simulink model "WF_status"  (R2022b)
settings: Solver=FixedStepDiscrete  StartTime=0  StopTime=duration  FixedStep=sample_time  RelTol=1e-3
values from neighbouring files (symbols this model uses):
  WF_status_param =     [WF_status_params.mat]
libraries: simulink x6
settings Model: Creator=Carlo_TUM  LastModifiedBy=Carlo_TUM
settings DataIOCC: LoadExternalInput=on  ReturnWorkspaceOutputs=off  ReturnWorkspaceOutputsName=off
settings OptimizationCC: DefaultParameterBehavior=Inlined  EnhancedBackFolding=on  PassReuseOutputArgsAs=Individual arguments  OptimizeBlockOrder=speed  DifferentSizesBufferReuse=on  OptimizationCustomize=off  EfficientTunableParamExpr=on
settings DebuggingCC: ParameterTunabilityLossMsg=error
settings SFSimCC: MATLABDynamicMemAlloc=off
settings RTWCC: Description=Embedded Coder  SystemTargetFile=ert.tlc  TemplateMakefile=ert_default_tmf
settings CodeAppCC: ForceParamTrailComments=on  IgnoreCustomStorageClasses=off  OperatorAnnotations=on  SimulinkDataObjDesc=on  SFDataObjDesc=on  InsertBlockDesc=on
settings ERTTargetCC: TargetLangStandard=C99 (ISO)  GenerateSampleERTMain=on  InlinedParameterPlacement=NonHierarchical  ERTCustomFileTemplate=example_file_process.tlc

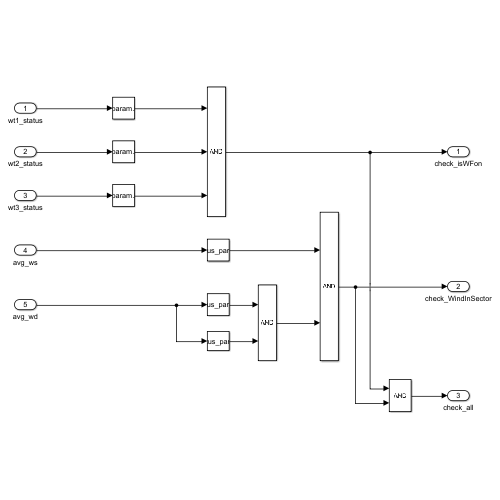
[thumbnail: Simulink's stored preview of the top-level diagram]
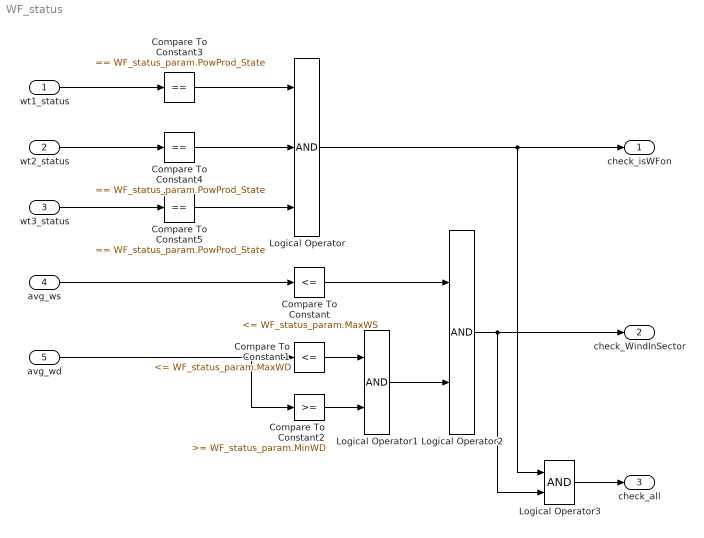
== system WF_status ==
  wt1_status : Inport
  wt2_status : Inport  Port=2
  wt3_status : Inport  Port=3
  avg_ws : Inport  Port=4
  avg_wd : Inport  Port=5
  Compare To Constant : simulink/Logic and Bit Operations/Compare To Constant  relop=<=  const=WF_status_param.MaxWS  OutDataTypeStr=boolean
  Compare To Constant1 : simulink/Logic and Bit Operations/Compare To Constant  relop=<=  const=WF_status_param.MaxWD  OutDataTypeStr=boolean
  Compare To Constant2 : simulink/Logic and Bit Operations/Compare To Constant  relop=>=  const=WF_status_param.MinWD  OutDataTypeStr=boolean
  Compare To Constant3 : simulink/Logic and Bit Operations/Compare To Constant  relop===  const=WF_status_param.PowProd_State  OutDataTypeStr=boolean
  Compare To Constant4 : simulink/Logic and Bit Operations/Compare To Constant  relop===  const=WF_status_param.PowProd_State  OutDataTypeStr=boolean
  Compare To Constant5 : simulink/Logic and Bit Operations/Compare To Constant  relop===  const=WF_status_param.PowProd_State  OutDataTypeStr=boolean
  Logical Operator : Logic  Inputs=3  AllPortsSameDT=off  OutDataTypeStr=boolean
  Logical Operator1 : Logic  AllPortsSameDT=off  OutDataTypeStr=boolean
  Logical Operator2 : Logic  AllPortsSameDT=off  OutDataTypeStr=boolean
  Logical Operator3 : Logic  AllPortsSameDT=off  OutDataTypeStr=boolean
  check_isWFon : Outport
  check_WindInSector : Outport  Port=2
  check_all : Outport  Port=3
  wires:
  wt1_status/1 -> Compare To Constant3/1
  wt2_status/1 -> Compare To Constant4/1
  wt3_status/1 -> Compare To Constant5/1
  Logical Operator/1 -> Logical Operator3/1, check_isWFon/1
  avg_ws/1 -> Compare To Constant/1
  avg_wd/1 -> Compare To Constant2/1, Compare To Constant1/1
  Compare To Constant1/1 -> Logical Operator1/1
  Compare To Constant/1 -> Logical Operator2/1
  Compare To Constant2/1 -> Logical Operator1/2
  Logical Operator1/1 -> Logical Operator2/2
  Logical Operator2/1 -> Logical Operator3/2, check_WindInSector/1
  Logical Operator3/1 -> check_all/1
  Compare To Constant3/1 -> Logical Operator/1
  Compare To Constant4/1 -> Logical Operator/2
  Compare To Constant5/1 -> Logical Operator/3
